simulink model "smceso_simscape"  (R2024a)
settings: Solver=VariableStepAuto  StartTime=0.0  StopTime=150  FixedStep=0.05  RelTol=1e-3  AbsTol=1e-3  EnableMultiTasking=on
model workspace (MATLAB code in the model file):
  | rCord = 0.25; % Cord radius, in
  | rho = 8000; % Density (steel), kg/m^3
  | 
  | % Hoist Pulleys:
  | rContactHoist = 7; % Contact radius, in
  | rPitchHoist = rContactHoist + rCord; % Pitch radius, in
  | Hoist.RGB = [0.35 0.35 1.0]; % Color, RGB 0-1
  | 
  | % Trolley Pulleys:
  | rContactTrolley = 5; % Contact radius, in
  | rPitchTrolley = rContactTrolley + rCord; % Pitch radius, in
  | Trolley.RGB = [1 0.15 0.15]; % Color, RGB 0-1
values from neighbouring files (symbols this model uses):
  m = 500    [finiteeso1.m]    (also in myIneqConFunction.m; robot_model.m)
  s = dq1 + lambda*(q1-q1d) + alpha*q2    [myIneqConFunction.m]
undefined symbols (not defined in the file or in its folder): X, Y, Z
libraries: sm_lib x19, nesl_utility x10
CloseFcn:
  | try,close(h1_sm_cable_tower_crane),end
  | clear h1_sm_cable_tower_crane
  | 
  | clear simlog_sm_cable_tower_crane
  | clear logsout_sm_cable_tower_crane
Description:
  | Tower Crane With Trolley and Hoist
settings Model: Creator=The MathWorks, Inc.  LastModifiedBy=vanch
settings SolverCC: AutoInsertRateTranBlk=on
settings DataIOCC: MaxDataPoints=10000  ReturnWorkspaceOutputs=off  SignalLoggingName=logsout_sm_cable_tower_crane
settings OptimizationCC: LifeSpan=inf
settings DebuggingCC: MultiTaskRateTransMsg=warning  UnconnectedInputMsg=warning  UnconnectedOutputMsg=warning  UnconnectedLineMsg=warning  AllowSymbolicDim=off  PregeneratedLibrarySubsystemCodeDiagnostic=none  SFUnexpectedBacktrackingDiag=warning  SFNoUnconditionalDefaultTransitionDiag=warning  SFExecutionAtInitializationDiag=none  ArithmeticOperatorsInVariantConditions=warning
settings ModelReferenceCC: EnableRefExpFcnMdlSchedulingChecks=on
settings SFSimCC: SimUseLocalCustomCode=off  CustomCodeUndefinedFunction=UseInterfaceOnly
settings RTWCC: RTWUseLocalCustomCode=off  GPUComputeCapability=3.5  DLArmComputeVersion=19.05
settings CodeAppCC: StateflowObjectComments=on
settings GRTTargetCC: TargetLangStandard=C89/C90 (ANSI)
settings ConfigComp: CovMetricSettings=dw  CovSaveCumulativeToWorkspaceVar=on  CovSaveSingleToWorkspaceVar=on  CovExternalEMLEnable=off  CovSFcnEnable=off
settings SimscapeCC: SimscapeNormalizeSystem=off  SimscapeLogType=all  SimscapeLogSimulationStatistics=on  SimscapeLogName=simlog_sm_cable_tower_crane  SimscapeLogDataHistory=10000
settings ConfigurationSet: Description=SimMechanics 2G
settings DiagnosticsConfigSet: SimMechanicsUnconnectedFramePorts=none
settings ExplorerConfigSet: InternalSimMechanicsExplorerSettings="<ExplorerConfiguration><canonicalview>default</canonicalview><AnimationSetting><BasePlaybackSpeed>1.0</BasePlaybackSpeed><PlaybackSpeedFactor>4.0</PlaybackSpeedFactor></AnimationSetting><TilePanel><TileInfo><Tiles Columns=\"2\" Count=\"3\" Rows=\"2\"><Column Weight=\"0.5346\"/><Column Weight=\"0.4654\"/><Row Weight=\"0.5103\"/><Row Weight=\"0.4897\"/><Tile Height=\"2\" Width=\"1\" X=\"0\" Y=\"0\"/><Tile Height=\"1\" Width=\"1\" X=\"1\" Y=\"0\"/><Tile Height=\"1\" Width=\"1\" X=\"1\" Y=\"1\"/></Tiles></TileInfo><SceneInfo><SceneViewer><BGColor><R>1</R><G>1</G><B>1</B></BGColor><Camera><DoPerspective>off</DoPerspective><Position><X>21.2245234512222218</X><Y>-52.6270053119242149</Y><Z>31.1052414476314176</Z></Position><Center><X>4.03969410390390138</X><Y>-11.531029179114606</Y><Z>26.0581003831327429</Z></Center><Up><X>-0.0463963572767632781</X><Y>0.102630781540790306</Y><Z>0.993636905872448795</Z></Up><ViewLimDist>1</ViewLimDist><YLim>29.3741015052795404</YLim><XLim>20.323349428569383</XLim></Camera></SceneViewer><SceneViewer><BGColor><R>1</R><G>1</G><B>1</B></BGColor><Camera><DoPerspective>on</DoPerspective><Position><X>7.62097636835298875</X><Y>-7.28765998656097835</Y><Z>48.5790735257936888</Z></Position><Center><X>8.43815474417762879</X><Y>-4.87266112484600811</Y><Z>48.0790735257936888</Z></Center><Up><X>-5.5511151231257827e-17</X><Y>5.5511151231257827e-16</Y><Z>1</Z></Up><ViewLimDist>1</ViewLimDist><YLim>0.466307658154998583</YLim><XLim>0.554639064765857337</XLim></Camera></SceneViewer><SceneViewer><BGColor><R>1</R><G>1</G><B>1</B></BGColor><Camera><DoPerspective>on</DoPerspective><Position><X>8.91771748690350918</X><Y>-5.72696404215155486</Y><Z>6.27537931293847695</Z></Position><Center><X>8.30176786249526799</X><Y>-4.79390373339482956</Y><Z>6.27750543949919315</Z></Center><Up><X>0.0018411954977133882</X><Y>-0.00106320895941669491</Y><Z>0.999997739790369544</Z></Up><ViewLimDist>1</ViewLimDist><YLim>0.466307658154998583</YLim><XLim>0.577537007806649627</XLim></Camera></SceneViewer></SceneInfo></TilePanel><MechEditorPanel><Cameras><Camera><Id>Camera3</Id><Value><Name>FrontPerspective</Name><NativeCamera><PositionKeyframeSet><Keyframe><Time>+0.0000000000000000e+00</Time><Value><X>-8.2854741987599496e+01</X><Y>+6.9234458953745950e+00</Y><Z>-1.4145124864096545e+01</Z></Value></Keyframe></PositionKeyframeSet><CenterKeyframeSet><Keyframe><Time>+0.0000000000000000e+00</Time><Value><X>-3.8386611818308438e+01</X><Y>+5.6305115971696154e+00</Y><Z>-1.4885098486593563e+01</Z></Value></Keyframe></CenterKeyframeSet><UpVectorKeyframeSet><Keyframe><Time>+0.0000000000000000e+00</Time><Value><X>+1.6618412601474140e-02</X><Y>-6.8180478671186931e-04</Y><Z>+9.9986167218512778e-01</Z></Value></Keyframe></UpVectorKeyframeSet></NativeCamera></Value></Camera><Camera><Id>Camera4</Id><Value><Name>IsoPerspective</Name><NativeCamera><PositionKeyframeSet><Keyframe><Time>+0.0000000000000000e+00</Time><Value><X>+4.8041868307394381e+01</X><Y>-7.2574542010436318e+01</Y><Z>-1.9623596137357460e+01</Z></Value></Keyframe></PositionKeyframeSet><CenterKeyframeSet><Keyframe><Time>+0.0000000000000000e+00</Time><Value><X>+1.8405017763935820e+01</X><Y>-3.4347633911723840e+01</Y><Z>-1.7683820531547433e+01</Z></Value></Keyframe></CenterKeyframeSet><UpVectorKeyframeSet><Keyframe><Time>+0.0000000000000000e+00</Time><Value><X>+2.6442579825491388e-02</X><Y>-3.0202215803021151e-02</Y><Z>+9.9919398323486741e-01</Z></Value></Keyframe></UpVectorKeyframeSet></NativeCamera></Value></Camera><Camera><Id>Camera5</Id><Value><Name>TrolleyCam</Name><NativeCamera><PositionTrackingFeature>Tower_Crane.Trolley.Transform_Trolley_Cam.F</PositionTrackingFeature><CenterTrackingFeature>Tower_Crane.Trolley.Trolley.R</CenterTrackingFeature><UpVectorTrackingFeature>Tower_Crane.Trolley.Trolley.R</UpVectorTrackingFeature><CenterTrackingOrigin>on</CenterTrackingOrigin><UpVectorTrackingDirection>+Y</UpVectorTrackingDirection></NativeCamera></Value></Camera><Camera><Id>Camera6</Id><Value><Name>BlockCam</Name><NativeCamera><PositionTrackingFeature>Tower_Crane.Hoist_Pulleys.Transform_Block_Cam.F</PositionTrackingFeature><CenterTrackingFeature>Tower_Crane.Hoist_Pulleys.Revolute_Block_Pulley.F</CenterTrackingFeature><UpVectorTrackingFeature>Tower_Crane.Hoist_Pulleys.Revolute_Block_Pulley.F</UpVectorTrackingFeature><CenterTrackingOrigin>on</CenterTrackingOrigin><UpVectorTrackingDirection>-Y</UpVectorTrackingDirection></NativeCamera></Value></Camera></Cameras><GfxPanelCameraMap><MapElement CameraMLId=\"Camera5\" GfxPanelIndex=\"1\"/><MapElement CameraMLId=\"Camera6\" GfxPanelIndex=\"2\"/></GfxPanelCameraMap><VideoCreator><PlaybackSpeedRatio>1.0</PlaybackSpeedRatio><FrameRate>30</FrameRate><VideoFormat>MPEG-4</VideoFormat><FrameSize>auto</FrameSize></VideoCreator></MechEditorPanel></ExplorerConfiguration>"

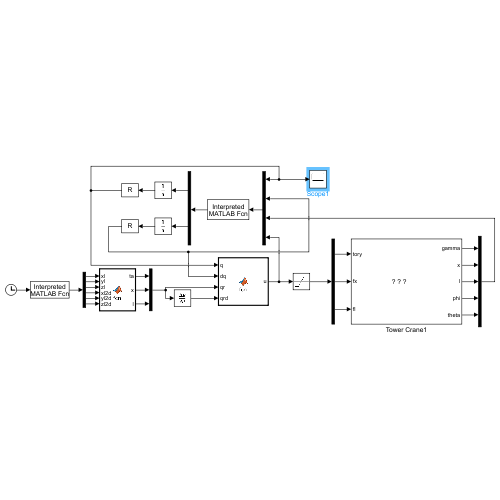
[thumbnail: Simulink's stored preview of the top-level diagram]
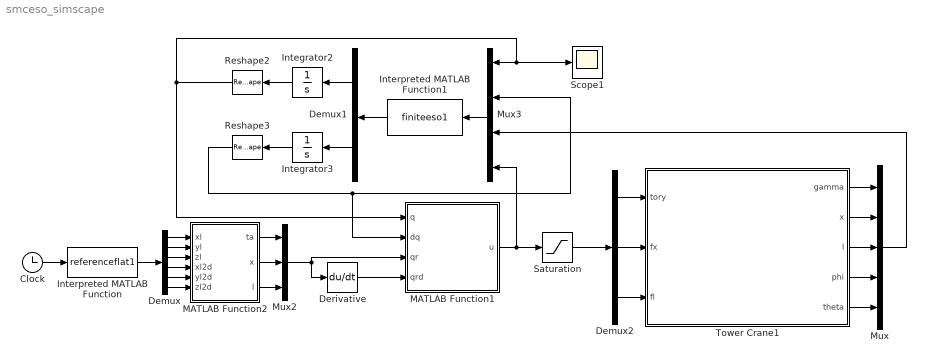
== system smceso_simscape ==
  Clock : Clock
  Demux : Demux  Outputs=6
  Demux1 : Demux  Outputs=2
  Demux2 : Demux  Outputs=3
  Derivative : Derivative
  Integrator2 : Integrator  InitialCondition=[0;0;45;0;0]
  Integrator3 : Integrator  InitialCondition=[0;0;0;0;0]
  Interpreted MATLAB Function : MATLABFcn  MATLABFcn=referenceflat1  OutputDimensions=6
  Interpreted MATLAB Function1 : MATLABFcn  MATLABFcn=finiteeso1
  MATLAB Function1 : MATLAB Function  TreatAsAtomicUnit=on
  MATLAB Function2 : MATLAB Function  TreatAsAtomicUnit=on
  Mux : Mux  Inputs=5
  Mux2 : Mux  Inputs=3
  Mux3 : Mux
  Reshape2 : Reshape  OutputDimensionality=Customize  OutputDimensions=[5,1]
  Reshape3 : Reshape  OutputDimensionality=Customize  OutputDimensions=[5,1]
  Saturation : Saturate  UpperLimit=[2000;400;0]  LowerLimit=[-2000;-400;-6000]
  Scope1 : Scope
  Tower Crane1 : Subsystem  Tag=PublishSubsystem
      mask Display: image('sm_cable_tower_crane_all_IMAGE.png');
  wires:
  Demux2/1 -> Tower Crane1/1(tory)
  Demux2/2 -> Tower Crane1/2(fx)
  Demux2/3 -> Tower Crane1/3(fl)
  Clock/1 -> Interpreted MATLAB Function/1
  Mux2/1 -> Derivative/1, MATLAB Function1/3(qr)
  MATLAB Function2/1(ta) -> Mux2/1
  Mux/1 -> Mux3/3
  Demux/4 -> MATLAB Function2/4(xl2d)
  Demux/3 -> MATLAB Function2/3(zl)
  Mux3/1 -> Interpreted MATLAB Function1/1
  Demux1/2 -> Integrator3/1
  Derivative/1 -> MATLAB Function1/4(qrd)
  MATLAB Function2/2(x) -> Mux2/2
  Interpreted MATLAB Function/1 -> Demux/1
  Integrator2/1 -> Reshape2/1
  Reshape3/1 -> Mux3/2, MATLAB Function1/2(dq)
  Integrator3/1 -> Reshape3/1
  Interpreted MATLAB Function1/1 -> Demux1/1
  Reshape2/1 -> Scope1/1, Mux3/1, MATLAB Function1/1(q)
  Demux/5 -> MATLAB Function2/5(yl2d)
  MATLAB Function2/3(l) -> Mux2/3
  Demux/6 -> MATLAB Function2/6(zl2d)
  Demux/1 -> MATLAB Function2/1(xl)
  MATLAB Function1/1(u) -> Saturation/1, Mux3/4
  Demux/2 -> MATLAB Function2/2(yl)
  Demux1/1 -> Integrator2/1
  Tower Crane1/1(gamma) -> Mux/1
  Tower Crane1/2(x) -> Mux/2
  Tower Crane1/3(l) -> Mux/3
  Tower Crane1/4(phi) -> Mux/4
  Tower Crane1/5(theta) -> Mux/5
  Saturation/1 -> Demux2/1

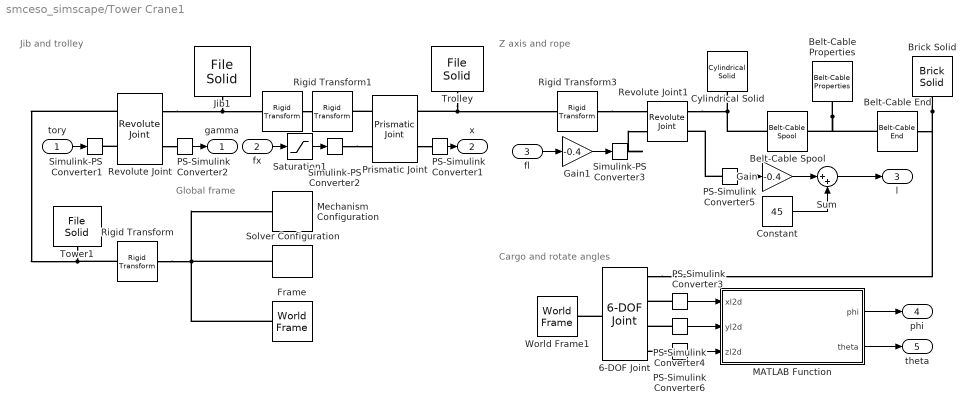
== system smceso_simscape/Tower Crane1 ==
  note: Z axis and rope
  note: Cargo and rotate
      | angles
  note: Jib and trolley
  note: Global frame
  tory : Inport
  fx : Inport  Port=2
  fl : Inport  Port=3
  " Frame" : sm_lib/Frames and Transforms/World Frame
  " " : sm_lib/Frames and Transforms/Rigid Transform  RotationMethod=StandardAxis  FollAlignAxisA=+X  BaseAlignAxisA=+Y  FollAlignAxisB=+Y  BaseAlignAxisB=+Z  RotationStandardAxis=+X  RotationAngle=90  RotationAngleUnits=deg  RotationArbitraryAxis=[0 0 1]  RotationSequenceAxes=FollowerAxes  RotationSequence=XYX  RotationSequenceAngles=[0 0 0]  RotationSequenceAnglesUnits=deg  RotationMatrix=[1 0 0; 0 1 0; 0 0 1]  Quaternion=[1 0 0 0]  TranslationMethod=StandardAxis  TranslationCartesianOffset=[-2.5 0.5 0.5]  TranslationCartesianOffsetUnits=m  TranslationStandardAxis=+Y  TranslationStandardOffset=3.2  TranslationStandardOffsetUnits=m  TranslationROffset=0  TranslationROffsetUnits=m  TranslationThetaOffset=0  TranslationThetaOffsetUnits=deg  TranslationZOffset=0  TranslationZOffsetUnits=m
  6-DOF Joint : sm_lib/Joints/6-DOF Joint  JointMode=Normal  CompositeWrenchDir=FollowerOnBase  CompositeWrenchFrame=BaseFrame  SenseConstraintForce=off  SenseConstraintTorque=off  SenseTotalForce=off  SenseTotalTorque=off  PxPositionTargetSpecify=on  PxPositionTargetPriority=High  PxPositionTargetValue=-6  PxPositionTargetValueUnits=m  PxVelocityTargetSpecify=off  PxVelocityTargetPriority=High  PxVelocityTargetValue=0  PxVelocityTargetValueUnits=m/s  PxEquilibriumPosition=0  PxEquilibriumPositionUnits=m  PxSpringStiffness=0  PxSpringStiffnessUnits=N/m  PxDampingCoefficient=0  PxDampingCoefficientUnits=N/(m/s)  PxLowerLimitSpecify=off  PxLowerLimitBound=-1  PxLowerLimitBoundUnits=m  PxLowerLimitStiffness=1e6  PxLowerLimitStiffnessUnits=N/m  PxLowerLimitDamping=1e3  PxLowerLimitDampingUnits=N/(m/s)  PxLowerLimitTransitionRegionWidth=1e-4  PxLowerLimitTransitionRegionWidthUnits=m  PxUpperLimitSpecify=off  PxUpperLimitBound=1  PxUpperLimitBoundUnits=m  PxUpperLimitStiffness=1e6  PxUpperLimitStiffnessUnits=N/m  PxUpperLimitDamping=1e3  PxUpperLimitDampingUnits=N/(m/s)  PxUpperLimitTransitionRegionWidth=1e-4  PxUpperLimitTransitionRegionWidthUnits=m  PxTorqueActuationMode=NoTorque  PxMotionActuationMode=ComputedMotion  PxSensePosition=off  PxSenseVelocity=off  PxSenseAcceleration=on  PxSenseTorqueForce=off  PxSenseLowerLimitTorqueForce=off  PxSenseUpperLimitTorqueForce=off  PyPositionTargetSpecify=on  PyPositionTargetPriority=High  PyPositionTargetValue=0  PyPositionTargetValueUnits=m  PyVelocityTargetSpecify=off  PyVelocityTargetPriority=High  PyVelocityTargetValue=0  PyVelocityTargetValueUnits=m/s  PyEquilibriumPosition=0  PyEquilibriumPositionUnits=m  PySpringStiffness=0  PySpringStiffnessUnits=N/m  PyDampingCoefficient=0  PyDampingCoefficientUnits=N/(m/s)  PyLowerLimitSpecify=off  PyLowerLimitBound=-1  PyLowerLimitBoundUnits=m  PyLowerLimitStiffness=1e6  PyLowerLimitStiffnessUnits=N/m  PyLowerLimitDamping=1e3  PyLowerLimitDampingUnits=N/(m/s)  PyLowerLimitTransitionRegionWidth=1e-4  PyLowerLimitTransitionRegionWidthUnits=m  PyUpperLimitSpecify=off  PyUpperLimitBound=1  PyUpperLimitBoundUnits=m  PyUpperLimitStiffness=1e6  PyUpperLimitStiffnessUnits=N/m  PyUpperLimitDamping=1e3  PyUpperLimitDampingUnits=N/(m/s)  PyUpperLimitTransitionRegionWidth=1e-4  PyUpperLimitTransitionRegionWidthUnits=m  PyTorqueActuationMode=NoTorque  PyMotionActuationMode=ComputedMotion  PySensePosition=off  PySenseVelocity=off  PySenseAcceleration=on  PySenseTorqueForce=off  PySenseLowerLimitTorqueForce=off  PySenseUpperLimitTorqueForce=off  PzPositionTargetSpecify=on  PzPositionTargetPriority=High  PzPositionTargetValue=3  PzPositionTargetValueUnits=m  PzVelocityTargetSpecify=off  PzVelocityTargetPriority=High  PzVelocityTargetValue=0  PzVelocityTargetValueUnits=m/s  PzEquilibriumPosition=0  PzEquilibriumPositionUnits=m  PzSpringStiffness=0  PzSpringStiffnessUnits=N/m  PzDampingCoefficient=30  PzDampingCoefficientUnits=N/(m/s)  PzLowerLimitSpecify=off  PzLowerLimitBound=-1  PzLowerLimitBoundUnits=m  PzLowerLimitStiffness=1e6  PzLowerLimitStiffnessUnits=N/m  PzLowerLimitDamping=1e3  PzLowerLimitDampingUnits=N/(m/s)  PzLowerLimitTransitionRegionWidth=1e-4  PzLowerLimitTransitionRegionWidthUnits=m  PzUpperLimitSpecify=off  PzUpperLimitBound=1  PzUpperLimitBoundUnits=m  PzUpperLimitStiffness=1e6  PzUpperLimitStiffnessUnits=N/m  PzUpperLimitDamping=1e3  PzUpperLimitDampingUnits=N/(m/s)  PzUpperLimitTransitionRegionWidth=1e-4  PzUpperLimitTransitionRegionWidthUnits=m  PzTorqueActuationMode=NoTorque  PzMotionActuationMode=ComputedMotion  PzSensePosition=off  PzSenseVelocity=off  PzSenseAcceleration=on  PzSenseTorqueForce=off  PzSenseLowerLimitTorqueForce=off  PzSenseUpperLimitTorqueForce=off  SphPositionTargetSpecify=off  SphPositionTargetPriority=High  SphPositionTargetRotationMethod=None  SphPositionTargetFollAlignAxisA=+X  SphPositionTargetBaseAlignAxisA=+Y  SphPositionTargetFollAlignAxisB=+Y  SphPositionTargetBaseAlignAxisB=+Z  SphPositionTargetRotationStandardAxis=+Z  SphPositionTargetRotationAngle=0.0  SphPositionTargetRotationAngleUnits=deg  SphPositionTargetRotationArbitraryAxis=[0 0 1]  SphPositionTargetRotationSequenceAxes=FollowerAxes  SphPositionTargetRotationSequence=XYX  SphPositionTargetRotationSequenceAngles=[0 0 0]  SphPositionTargetRotationSequenceAnglesUnits=deg  SphPositionTargetRotationMatrix=[1 0 0; 0 1 0; 0 0 1]  SphPositionTargetQuaternion=[1 0 0 0]  SphVelocityTargetSpecify=off  SphVelocityTargetPriority=High  SphVelocityTargetValue=[0 0 0]  SphVelocityTargetValueUnits=deg/s  SphVelocityTargetInFollowerFrame=on  SphEqPosRotationMethod=None  SphEqPosFollAlignAxisA=+X  SphEqPosBaseAlignAxisA=+Y  SphEqPosFollAlignAxisB=+Y  SphEqPosBaseAlignAxisB=+Z  SphEqPosRotationStandardAxis=+Z  SphEqPosRotationAngle=0.0  SphEqPosRotationAngleUnits=deg  SphEqPosRotationArbitraryAxis=[0 0 1]  SphEqPosRotationSequenceAxes=FollowerAxes  SphEqPosRotationSequence=XYX  SphEqPosRotationSequenceAngles=[0 0 0]  SphEqPosRotationSequenceAnglesUnits=deg  SphEqPosRotationMatrix=[1 0 0; 0 1 0; 0 0 1]  SphEqPosQuaternion=[1 0 0 0]  SphSpringStiffness=0  SphSpringStiffnessUnits=N*m/deg  SphDampingCoefficient=0  SphDampingCoefficientUnits=N*m/(deg/s)  SphLowerLimitSpecify=off  SphLowerLimitBound=15  SphLowerLimitBoundUnits=deg  SphLowerLimitStiffness=1e4  SphLowerLimitStiffnessUnits=N*m/deg  SphLowerLimitDamping=10  SphLowerLimitDampingUnits=N*m/(deg/s)  SphLowerLimitTransitionRegionWidth=0.1  SphLowerLimitTransitionRegionWidthUnits=deg  SphUpperLimitSpecify=off  SphUpperLimitBound=45  SphUpperLimitBoundUnits=deg  SphUpperLimitStiffness=1e4  SphUpperLimitStiffnessUnits=N*m/deg  SphUpperLimitDamping=10  SphUpperLimitDampingUnits=N*m/(deg/s)  SphUpperLimitTransitionRegionWidth=0.1  SphUpperLimitTransitionRegionWidthUnits=deg  SphTorqueActuationMode=NoTorque  SphActuateTorqueX=off  SphActuateTorqueY=off  SphActuateTorqueZ=off  SphActuateTorque=off  SphActuationFrame=BaseFrame  SphSensePosition=off  SphSenseVelocityX=off  SphSenseVelocityY=off  SphSenseVelocityZ=off  SphSenseVelocity=off  SphSenseAccelerationX=off  SphSenseAccelerationY=off  SphSenseAccelerationZ=off  SphSenseAcceleration=off  SphSenseLowerLimitTorqueMag=off  SphSenseUpperLimitTorqueMag=off  SphSensingFrame=BaseFrame
  Belt-Cable Properties : sm_lib/Belts and Cables/Belt-Cable Properties  DrumBeltCableAlignment=Unrestricted  GraphicType=PitchLine  GraphicVisPropType=SimpleVisualProperties  GraphicDiffuseColor=[0.5 0.5 0.5]  GraphicOpacity=1.0  GraphicSpecularColor=[0.5 0.5 0.5 1.0]  GraphicAmbientColor=[0.15 0.15 0.15 1.0]  GraphicEmissiveColor=[0.0 0.0 0.0 1.0]  GraphicShininess=75
  Belt-Cable End : sm_lib/Belts and Cables/Belt-Cable End
  Belt-Cable Spool : sm_lib/Belts and Cables/Belt-Cable Spool  PitchRadius=0.4  PitchRadiusUnits=m  SenseSpoolAngleA=off  SenseFleetAngleA=off
  Brick Solid : sm_lib/Body Elements/Brick Solid  BrickDimensions=[1 1 1]  BrickDimensionsUnits=m  ExportEntireGeometry=off  InertiaType=CalculateFromGeometry  BasedOnType=Density  Density=500  DensityUnits=kg/m^3  Mass=1  MassUnits=kg  CenterOfMass=[0 0 0]  CenterOfMassUnits=m  MomentsOfInertia=[1 1 1]  MomentsOfInertiaUnits=kg*m^2  ProductsOfInertia=[0 0 0]  ProductsOfInertiaUnits=kg*m^2  GraphicType=FromGeometry  MarkerShape=Sphere  MarkerSize=10  GraphicVisPropType=SimpleVisualProperties  GraphicDiffuseColor=[0.5 0.5 0.5]  GraphicOpacity=1.0  GraphicSpecularColor=[0.5 0.5 0.5 1.0]  GraphicAmbientColor=[0.15 0.15 0.15 1.0]  GraphicEmissiveColor=[0.0 0.0 0.0 1.0]  GraphicShininess=75  DoExposeReferenceFrame=on  SerializedFrames=<Frames/>
  Constant : Constant  Value=45
  Cylindrical Solid : sm_lib/Body Elements/Cylindrical Solid  CylinderRadius=0.5  CylinderRadiusUnits=m  CylinderLength=0.4  CylinderLengthUnits=m  ExportEntireGeometry=off  InertiaType=CalculateFromGeometry  BasedOnType=Density  Density=1000  DensityUnits=kg/m^3  Mass=1  MassUnits=kg  CenterOfMass=[0 0 0]  CenterOfMassUnits=m  MomentsOfInertia=[1 1 1]  MomentsOfInertiaUnits=kg*m^2  ProductsOfInertia=[0 0 0]  ProductsOfInertiaUnits=kg*m^2  GraphicType=FromGeometry  MarkerShape=Sphere  MarkerSize=10  GraphicVisPropType=SimpleVisualProperties  GraphicDiffuseColor=[0.5 0.5 0.5]  GraphicOpacity=1.0  GraphicSpecularColor=[0.5 0.5 0.5 1.0]  GraphicAmbientColor=[0.15 0.15 0.15 1.0]  GraphicEmissiveColor=[0.0 0.0 0.0 1.0]  GraphicShininess=75  DoExposeReferenceFrame=on  SerializedFrames=<Frames/>
  Gain : Gain  Gain=-0.4
  Gain1 : Gain  Gain=-0.4
  Jib1 : sm_lib/Body Elements/File Solid  ExtGeomFileName=jib.step  UnitType=FromFile  ExtGeomFileUnits=m  StepReaderType=HEX  ExportConvexHullGeometry=off  InertiaType=CalculateFromGeometry  BasedOnType=Density  Density=400  DensityUnits=kg/(m^3)  Mass=1  MassUnits=kg  CenterOfMass=[0 0 0]  CenterOfMassUnits=m  MomentsOfInertia=[1 1 1]  MomentsOfInertiaUnits=kg*m^2  ProductsOfInertia=[0 0 0]  ProductsOfInertiaUnits=kg*m^2  GraphicType=FromGeometry  MarkerShape=Sphere  MarkerSize=10  GraphicVisPropType=AdvancedVisualProperties  GraphicDiffuseColor=[0.15 0.15 0.15]  GraphicOpacity=1.0  GraphicSpecularColor=[0.6 0.6 0.6]  GraphicAmbientColor=[0.1 0.1 0.1]  GraphicEmissiveColor=[0.0 0.0 0.0 1.0]  GraphicShininess=10  DoExposeReferenceFrame=on  SerializedFrames=<Frames/>
  MATLAB Function : MATLAB Function  TreatAsAtomicUnit=on
  Mechanism Configuration : sm_lib/Utilities/Mechanism Configuration  UniformGravity=Constant  GravityVector=[0 0 -9.81]  GravityVectorUnits=m/s^2  LinearizationDelta=0.001  JointModeTransitionNonlinearIterations=2
  PS-Simulink Converter{1..6} (6 alike) : nesl_utility/PS-Simulink Converter  PhysicalDomain=network_engine_domain  SubClassName=ps_output  LeftPortType=input  RightPortType=output  PseudoPeriodic=off  Frequencies=[]  VectorFormat=inherit  Unit=inherit  AffineConversion=off
  Prismatic Joint : sm_lib/Joints/Prismatic Joint  JointMode=Normal  CompositeWrenchDir=FollowerOnBase  CompositeWrenchFrame=BaseFrame  SenseConstraintForce=off  SenseConstraintTorque=off  SenseTotalForce=off  SenseTotalTorque=off  PositionTargetSpecify=off  PositionTargetPriority=High  PositionTargetValue=0  PositionTargetValueUnits=m  VelocityTargetSpecify=off  VelocityTargetPriority=High  VelocityTargetValue=0  VelocityTargetValueUnits=m/s  EquilibriumPosition=0  EquilibriumPositionUnits=m  SpringStiffness=0  SpringStiffnessUnits=N/m  DampingCoefficient=50  DampingCoefficientUnits=N/(m/s)  LowerLimitSpecify=off  LowerLimitBound=-1  LowerLimitBoundUnits=m  LowerLimitStiffness=1e6  LowerLimitStiffnessUnits=N/m  LowerLimitDamping=1e3  LowerLimitDampingUnits=N/(m/s)  LowerLimitTransitionRegionWidth=1e-4  LowerLimitTransitionRegionWidthUnits=m  UpperLimitSpecify=off  UpperLimitBound=1  UpperLimitBoundUnits=m  UpperLimitStiffness=1e6  UpperLimitStiffnessUnits=N/m  UpperLimitDamping=1e3  UpperLimitDampingUnits=N/(m/s)  UpperLimitTransitionRegionWidth=1e-4  UpperLimitTransitionRegionWidthUnits=m  TorqueActuationMode=InputTorque  MotionActuationMode=ComputedMotion  SensePosition=on  SenseVelocity=off  SenseAcceleration=off  SenseTorqueForce=off  SenseLowerLimitTorqueForce=off  SenseUpperLimitTorqueForce=off
  Revolute Joint : sm_lib/Joints/Revolute Joint  JointMode=Normal  CompositeWrenchDir=FollowerOnBase  CompositeWrenchFrame=BaseFrame  SenseConstraintForce=off  SenseConstraintTorque=off  SenseTotalForce=off  SenseTotalTorque=off  PositionTargetSpecify=off  PositionTargetPriority=High  PositionTargetValue=0  PositionTargetValueUnits=deg  VelocityTargetSpecify=off  VelocityTargetPriority=High  VelocityTargetValue=0  VelocityTargetValueUnits=deg/s  EquilibriumPosition=0  EquilibriumPositionUnits=deg  SpringStiffness=0  SpringStiffnessUnits=N*m/deg  DampingCoefficient=30  DampingCoefficientUnits=N*m/(deg/s)  LowerLimitSpecify=off  LowerLimitBound=-90  LowerLimitBoundUnits=deg  LowerLimitStiffness=1e4  LowerLimitStiffnessUnits=N*m/deg  LowerLimitDamping=10  LowerLimitDampingUnits=N*m/(deg/s)  LowerLimitTransitionRegionWidth=0.1  LowerLimitTransitionRegionWidthUnits=deg  UpperLimitSpecify=off  UpperLimitBound=90  UpperLimitBoundUnits=deg  UpperLimitStiffness=1e4  UpperLimitStiffnessUnits=N*m/deg  UpperLimitDamping=10  UpperLimitDampingUnits=N*m/(deg/s)  UpperLimitTransitionRegionWidth=0.1  UpperLimitTransitionRegionWidthUnits=deg  TorqueActuationMode=InputTorque  MotionActuationMode=ComputedMotion  SensePosition=on  SenseVelocity=off  SenseAcceleration=off  SenseTorqueForce=off  SenseLowerLimitTorqueForce=off  SenseUpperLimitTorqueForce=off
  Revolute Joint1 : sm_lib/Joints/Revolute Joint  JointMode=Normal  CompositeWrenchDir=FollowerOnBase  CompositeWrenchFrame=FollowerFrame  SenseConstraintForce=off  SenseConstraintTorque=off  SenseTotalForce=off  SenseTotalTorque=off  PositionTargetSpecify=off  PositionTargetPriority=High  PositionTargetValue=0  PositionTargetValueUnits=deg  VelocityTargetSpecify=off  VelocityTargetPriority=High  VelocityTargetValue=0  VelocityTargetValueUnits=deg/s  EquilibriumPosition=0  EquilibriumPositionUnits=deg  SpringStiffness=0  SpringStiffnessUnits=N*m/deg  DampingCoefficient=0  DampingCoefficientUnits=N*m/(deg/s)  LowerLimitSpecify=off  LowerLimitBound=-90  LowerLimitBoundUnits=deg  LowerLimitStiffness=1e4  LowerLimitStiffnessUnits=N*m/deg  LowerLimitDamping=10  LowerLimitDampingUnits=N*m/(deg/s)  LowerLimitTransitionRegionWidth=0.1  LowerLimitTransitionRegionWidthUnits=deg  UpperLimitSpecify=off  UpperLimitBound=90  UpperLimitBoundUnits=deg  UpperLimitStiffness=1e4  UpperLimitStiffnessUnits=N*m/deg  UpperLimitDamping=10  UpperLimitDampingUnits=N*m/(deg/s)  UpperLimitTransitionRegionWidth=0.1  UpperLimitTransitionRegionWidthUnits=deg  TorqueActuationMode=InputTorque  MotionActuationMode=ComputedMotion  SensePosition=on  SenseVelocity=off  SenseAcceleration=off  SenseTorqueForce=off  SenseLowerLimitTorqueForce=off  SenseUpperLimitTorqueForce=off
  Rigid Transform : sm_lib/Frames and Transforms/Rigid Transform  RotationMethod=None  FollAlignAxisA=+X  BaseAlignAxisA=+Y  FollAlignAxisB=+Y  BaseAlignAxisB=+Z  RotationStandardAxis=+Z  RotationAngle=0.0  RotationAngleUnits=deg  RotationArbitraryAxis=[0 0 1]  RotationSequenceAxes=FollowerAxes  RotationSequence=XYX  RotationSequenceAngles=[0 0 0]  RotationSequenceAnglesUnits=deg  RotationMatrix=[1 0 0; 0 1 0; 0 0 1]  Quaternion=[1 0 0 0]  TranslationMethod=StandardAxis  TranslationCartesianOffset=[0 0 0]  TranslationCartesianOffsetUnits=m  TranslationStandardAxis=+Z  TranslationStandardOffset=43.375  TranslationStandardOffsetUnits=m  TranslationROffset=0  TranslationROffsetUnits=m  TranslationThetaOffset=0  TranslationThetaOffsetUnits=deg  TranslationZOffset=0  TranslationZOffsetUnits=m
  Rigid Transform1 : sm_lib/Frames and Transforms/Rigid Transform  RotationMethod=StandardAxis  FollAlignAxisA=+X  BaseAlignAxisA=+Y  FollAlignAxisB=+Y  BaseAlignAxisB=+Z  RotationStandardAxis=-Y  RotationAngle=90  RotationAngleUnits=deg  RotationArbitraryAxis=[0 0 1]  RotationSequenceAxes=FollowerAxes  RotationSequence=XYX  RotationSequenceAngles=[0 0 0]  RotationSequenceAnglesUnits=deg  RotationMatrix=[1 0 0; 0 1 0; 0 0 1]  Quaternion=[1 0 0 0]  TranslationMethod=StandardAxis  TranslationCartesianOffset=[0 0 0]  TranslationCartesianOffsetUnits=m  TranslationStandardAxis=-X  TranslationStandardOffset=6  TranslationStandardOffsetUnits=m  TranslationROffset=0  TranslationROffsetUnits=m  TranslationThetaOffset=0  TranslationThetaOffsetUnits=deg  TranslationZOffset=0  TranslationZOffsetUnits=m
  Rigid Transform3 : sm_lib/Frames and Transforms/Rigid Transform  RotationMethod=StandardAxis  FollAlignAxisA=+X  BaseAlignAxisA=+Y  FollAlignAxisB=+Y  BaseAlignAxisB=+Z  RotationStandardAxis=+Z  RotationAngle=90  RotationAngleUnits=deg  RotationArbitraryAxis=[0 0 1]  RotationSequenceAxes=FollowerAxes  RotationSequence=XYX  RotationSequenceAngles=[0 0 0]  RotationSequenceAnglesUnits=deg  RotationMatrix=[1 0 0; 0 1 0; 0 0 1]  Quaternion=[1 0 0 0]  TranslationMethod=StandardAxis  TranslationCartesianOffset=[0 0 0]  TranslationCartesianOffsetUnits=m  TranslationStandardAxis=-Z  TranslationStandardOffset=0.4  TranslationStandardOffsetUnits=m  TranslationROffset=0  TranslationROffsetUnits=m  TranslationThetaOffset=0  TranslationThetaOffsetUnits=deg  TranslationZOffset=0  TranslationZOffsetUnits=m
  Saturation1 : Saturate  UpperLimit=100  LowerLimit=-100
  Simulink-PS Converter1 : nesl_utility/Simulink-PS Converter  PhysicalDomain=network_engine_domain  SubClassName=ps_input  LeftPortType=input  RightPortType=output  PseudoPeriodic=off  Frequencies=[]  NoiseDistribution=none  NoiseParameters=[]  Unit=1  AffineConversion=off  FilteringAndDerivatives=provide  SimscapeFilterOrder=1  InputFilterTimeConstant=0.001  UdotUserProvided=0
  Simulink-PS Converter2 : nesl_utility/Simulink-PS Converter  PhysicalDomain=network_engine_domain  SubClassName=ps_input  LeftPortType=input  RightPortType=output  PseudoPeriodic=off  Frequencies=[]  NoiseDistribution=none  NoiseParameters=[]  Unit=1  AffineConversion=off  FilteringAndDerivatives=provide  SimscapeFilterOrder=1  InputFilterTimeConstant=0.001  UdotUserProvided=0
  Simulink-PS Converter3 : nesl_utility/Simulink-PS Converter  PhysicalDomain=network_engine_domain  SubClassName=ps_input  LeftPortType=input  RightPortType=output  PseudoPeriodic=off  Frequencies=[]  NoiseDistribution=none  NoiseParameters=[]  Unit=1  AffineConversion=off  FilteringAndDerivatives=provide  SimscapeFilterOrder=1  InputFilterTimeConstant=0.001  UdotUserProvided=0
  Solver Configuration : nesl_utility/Solver Configuration  PhysicalDomain=network_engine_domain  SubClassName=solver  LeftPortType=input  RightPortType=generic  Tones=[]  Harmonics=[]  SimulateNoise=off  Profile=off  UseLocalSampling=off  EnableSwitchedLinearOptims=on  FrequencyDomain=off  UseCCode=off  RelTol=0.001  AbsTol=1e-06  MinStep=1e-09  ToWorkspace=off  RevertToSquareIcSolve=off  NumHomotopyIterations=100  PhasorMode=off  PhasorModeNumHarmonics=1  ConsistencySolver=NEWTON_FTOL  IndexReductionMethod=DerivativeReplacement  DoDC=off  ResidualTolerance=1e-09  ConsistencyTolSource=GLOBAL  ConsistencyAbsTol=0.001  ConsistencyRelTol=0.001  ConsistencyTolFactor=0.001  UseLocalSolver=off  LocalSolverChoice=NE_BACKWARD_EULER_ADVANCER  ResolveIndetEquations=on  FunctionEvalNumThread=1  LocalSolverSampleTime=0.001  DoFixedCost=off  MaxNonlinIter=3  MaxModeIter=2  ComputeImpulses=off  ImpulseIterations=1  LinearAlgebra=Sparse  LinearAlgebraNumThread=0  EquationFormulation=NE_TIME_EF  DelaysMemoryBudget=1024  AutomaticFiltering=on  FilteringTimeConstant=0.001  PartitionStorageMethod=AS_NEEDED  PartitionMemoryBudget=1024  PartitionMethod=FAST  MultibodyUseLocalSolver=off  MultibodyLocalSolverChoice=ODE1  MultibodyLocalSolverSampleTime=0.001
  Sum : Sum  Inputs=|++
  Tower1 : sm_lib/Body Elements/File Solid  ExtGeomFileName=tower.step  UnitType=FromFile  ExtGeomFileUnits=m  StepReaderType=HEX  ExportConvexHullGeometry=off  InertiaType=CalculateFromGeometry  BasedOnType=Density  Density=rho  DensityUnits=kg/(m^3)  Mass=1  MassUnits=kg  CenterOfMass=[0 0 0]  CenterOfMassUnits=m  MomentsOfInertia=[1 1 1]  MomentsOfInertiaUnits=kg*m^2  ProductsOfInertia=[0 0 0]  ProductsOfInertiaUnits=kg*m^2  GraphicType=FromGeometry  MarkerShape=Sphere  MarkerSize=10  GraphicVisPropType=AdvancedVisualProperties  GraphicDiffuseColor=[1.0 0.75 0.05]  GraphicOpacity=1.0  GraphicSpecularColor=[0.6 0.6 0.6]  GraphicAmbientColor=[0.1 0.1 0.1]  GraphicEmissiveColor=[0.0 0.0 0.0 1.0]  GraphicShininess=10  DoExposeReferenceFrame=on  SerializedFrames=<Frames/>
  "Trolley " : sm_lib/Body Elements/File Solid  ExtGeomFileName=trolley.step  UnitType=FromFile  ExtGeomFileUnits=m  StepReaderType=HEX  ExportConvexHullGeometry=off  InertiaType=CalculateFromGeometry  BasedOnType=Density  Density=7800  DensityUnits=kg/(m^3)  Mass=1  MassUnits=kg  CenterOfMass=[0 0 0]  CenterOfMassUnits=m  MomentsOfInertia=[1 1 1]  MomentsOfInertiaUnits=kg*m^2  ProductsOfInertia=[0 0 0]  ProductsOfInertiaUnits=kg*m^2  GraphicType=FromGeometry  MarkerShape=Sphere  MarkerSize=10  GraphicVisPropType=AdvancedVisualProperties  GraphicDiffuseColor=[1 0.75 0.05]  GraphicOpacity=1.0  GraphicSpecularColor=[0.4 0.4 0.4]  GraphicAmbientColor=[0 0 0]  GraphicEmissiveColor=[0 0 0]  GraphicShininess=10  DoExposeReferenceFrame=on  SerializedFrames=<Frames/>
  World Frame1 : sm_lib/Frames and Transforms/World Frame
  gamma : Outport
  x : Outport  Port=2
  l : Outport  Port=3
  phi : Outport  Port=4
  theta : Outport  Port=5
  wires:
  Gain1/1 -> Simulink-PS Converter3/1
  PS-Simulink Converter1/1 -> x/1
  PS-Simulink Converter2/1 -> gamma/1
  PS-Simulink Converter5/1 -> Gain/1
  fx/1 -> Saturation1/1
  Gain/1 -> Sum/1
  Sum/1 -> l/1
  Constant/1 -> Sum/2
  fl/1 -> Gain1/1
  tory/1 -> Simulink-PS Converter1/1
  Saturation1/1 -> Simulink-PS Converter2/1
  MATLAB Function/1(phi) -> phi/1
  MATLAB Function/2(theta) -> theta/1
  PS-Simulink Converter3/1 -> MATLAB Function/1(xl2d)
  PS-Simulink Converter4/1 -> MATLAB Function/2(yl2d)
  PS-Simulink Converter6/1 -> MATLAB Function/3(zl2d)
  connections:
  " "/LConn1 -- Rigid Transform1/LConn1
  Solver Configuration/RConn1 -- Mechanism Configuration/RConn1 -- Rigid Transform/LConn1 -- " Frame"/RConn1
  "Trolley "/RConn1 -- Prismatic Joint/RConn1 -- Rigid Transform3/LConn1
  Prismatic Joint/LConn1 -- Rigid Transform1/RConn1
  Simulink-PS Converter2/RConn1 -- Prismatic Joint/LConn2
  Tower1/RConn1 -- Revolute Joint/LConn1 -- Rigid Transform/RConn1
  Revolute Joint/LConn2 -- Simulink-PS Converter1/RConn1
  Jib1/RConn1 -- Revolute Joint/RConn1 -- " "/RConn1
  Belt-Cable Spool/LConn1 -- Revolute Joint1/RConn1 -- Cylindrical Solid/RConn1
  Brick Solid/RConn1 -- 6-DOF Joint/RConn1 -- Belt-Cable End/LConn1
  Belt-Cable Properties/LConn1 -- Belt-Cable End/RConn1 -- Belt-Cable Spool/RConn1
  Simulink-PS Converter3/RConn1 -- Revolute Joint1/LConn2
  Rigid Transform3/RConn1 -- Revolute Joint1/LConn1
  6-DOF Joint/LConn1 -- World Frame1/RConn1
  Prismatic Joint/RConn2 -- PS-Simulink Converter1/LConn1
  Revolute Joint/RConn2 -- PS-Simulink Converter2/LConn1
  PS-Simulink Converter5/LConn1 -- Revolute Joint1/RConn2
  PS-Simulink Converter3/LConn1 -- 6-DOF Joint/RConn2
  PS-Simulink Converter4/LConn1 -- 6-DOF Joint/RConn3
  PS-Simulink Converter6/LConn1 -- 6-DOF Joint/RConn4

== matlab function smceso_simscape/MATLAB Function1 ==
  data: q input; u output; dq input; qr input; qrd input
function u  = fcn(q, dq, qr,qrd)

mt=1140.7556;
j0=10215;
m=500;
bta=40;
bx=50;
bl=30;
btx=15;
bty=15;
g=9.81;

ta=q(1);
x=q(2);
l=q(3);
tx=q(4);
ty=q(5);
dta=dq(1);
dx=dq(2);
dl=dq(3);
dtx=dq(4);
dty=dq(5);
qa=[q(1);q(2);q(3)];
dqa=[dq(1);dq(2);dq(3)];
qu=[q(4);q(5)];
dqu=[dq(4);dq(5)];
e1=qa-qr;
e1d=dqa-qrd;
e2=[q(4);q(5)];

m11=j0+m*x^2+mt*x^2+m*l^2-m*l^2*cos(tx)^2*cos(ty)^2+2*m*x*l*cos(ty)*sin(tx);
m12=-m*l*sin(ty);
m13=m*x*sin(ty);
m14=-m*l^2*cos(tx)*cos(ty)*sin(ty);
m15=m*l^2*sin(tx)+m*x*l*cos(ty);
m21=-m*l*sin(ty);
m22=mt+m;
m23=m*cos(ty)*sin(tx);
m24=m*l*cos(tx)*cos(ty);
m25=-m*l*sin(tx)*sin(ty);
m31=m*x*sin(ty);
m32=m*cos(ty)*sin(tx);
m33=m;
m34=0;
m35=0;
m41=-m*l^2*cos(tx)*cos(ty)*sin(ty);
m42=m*l*cos(tx)*cos(ty);
m43=0;
m44=m*l^2*cos(ty)^2;
m45=0;
m51=m*l^2*sin(tx)+m*x*l*cos(ty);
m52=-m*l*sin(tx)*sin(ty);
m53=0;
m54=0;
m55=m*l^2;

c11=bta+m*x*dx+mt*x*dx+m*l*cos(ty)*sin(tx)*dx+m*l*dl-m*l*cos(tx)^2*cos(ty)^2*dl+m*x*cos(ty)*sin(tx)*dl+m*l^2*cos(tx)*cos(ty)^2*sin(tx)*dtx+m*l*x*cos(tx)*cos(ty)*dtx+m*l^2*cos(tx)^2*cos(ty)*sin(ty)*dty-m*x*l*sin(tx)*sin(ty)*dty;
c12=m*x*dta+mt*x*dta+m*l*cos(ty)*sin(tx)*dta;
c13=m*l*dta-m*l*cos(tx)^2*cos(ty)^2*dta+m*x*cos(ty)*sin(ty)*dta-m*l*cos(tx)*cos(ty)*sin(ty)*dtx+m*x*cos(ty)*dty+m*l*sin(tx)*dty;
c14=m*l^2*cos(tx)*cos(ty)^2*sin(ty)*dta+m*x*l*cos(tx)*cos(ty)*dta-m*l*cos(tx)*cos(ty)*sin(ty)*dl+m*l^2*cos(ty)*sin(tx)*sin(ty)*dtx+m*l^2*cos(tx)*dty-m*l^2*cos(tx)*cos(ty)^2*dty;
c15=m*l^2*cos(tx)^2*cos(ty)*sin(ty)*dta-m*x*l*sin(tx)*sin(ty)*dta+m*x*cos(ty)*dl+m*l*sin(tx)*dl+m*l^2*cos(tx)*dtx-m*l^2*cos(tx)*cos(ty)^2*dtx-m*x*l*sin(ty)*dty;
c21=-m*x*dta-mt*x*dta-m*l*cos(ty)*sin(tx)*dta-m*sin(ty)*dl-m*l*cos(ty)*dty;
c22=bx;
c23=-m*sin(ty)*dta+m*cos(tx)*cos(ty)*dtx-m*sin(tx)*sin(ty)*dty;
c24=m*cos(ty)*cos(tx)*dl-m*l*cos(ty)*sin(tx)*dtx-m*l*cos(tx)*sin(ty)*dty;
c25=-m*l*cos(ty)*dta-m*sin(tx)*sin(ty)*dl-m*l*cos(tx)*sin(ty)*dtx-m*l*cos(ty)*sin(tx)*dty;
c31=-m*l*dta+m*l*cos(tx)^2*cos(ty)^2*dta-m*x*cos(ty)*sin(tx)*dta+m*sin(ty)*dx+m*l*cos(tx)*cos(ty)*sin(ty)*dtx-m*l*sin(tx)*dty;
c32=m*sin(ty)*dta;
c33=bl;
c34=m*l*cos(tx)*cos(ty)*sin(ty)*dta-m*l*cos(ty)^2*dtx;
c35=-m*l*sin(tx)*dta-m*l*dty;
c41=-m*l^2*cos(tx)*cos(ty)^2*sin(tx)*dta-m*x*l*cos(tx)*cos(ty)*dta-m*l*cos(tx)*cos(ty)*sin(ty)*dl-m*l^2*cos(tx)*cos(ty)^2*dty;
c42=0;
c43=-m*l*cos(tx)*cos(ty)*sin(ty)*dta+m*l*cos(ty)^2*dtx;
c44=btx+m*l*cos(ty)^2*dl-m*l^2*cos(ty)*sin(ty)*dty;
c45=-m*l^2*cos(tx)*cos(ty)^2*dta-m*l^2*cos(ty)*sin(ty)*dtx;
c51=-m*l^2*cos(tx)^2*cos(ty)*sin(ty)*dta+m*l*x*sin(tx)*sin(ty)*dta+m*l*cos(ty)*dx+m*l*sin(tx)*dl+m*l^2*cos(tx)*cos(ty)^2*dtx;
c52=m*l*cos(ty)*dta;
c53=m*l*dty+m*l*sin(tx)*dta;
c54=m*l^2*cos(tx)*cos(ty)^2*dta+m*l^2*cos(ty)*sin(ty)*dtx;
c55=bty+m*l*dl;

g1=0;
g2=0;
g3=-m*g*cos(tx)*cos(ty);
g4=m*g*l*cos(ty)*sin(tx);
g5=m*g*l*cos(tx)*sin(ty);

M11=[m11 m12 m13;m21 m22 m23;m31 m32 m33];
M12=[m14 m15;m24 m25; m34 m35];
M21=[m41 m42 m43;m51 m52 m53];
M22=[m44 m45;m54 m55];
C11=[c11 c12 c13;c21 c22 c23;c31 c32 c33];
C12=[c14 c15;c24 c25; c34 c35];
C21=[c41 c42 c43;c51 c52 c53];
C22=[c44 c45;c54 c55];

G11=[g1;g2;g3];
G22=[g4;g5];

Mbar = M11 - M12*inv(M22)*M21;
C1bar = C11 - M12*inv(M22)*C21;
C2bar = C12 - M12*inv(M22)*C22;
Gbar = G11 - M12*inv(M22)*G22;

lamda1=0.75;
lamda2=0.5;
lamda3=0.85;
alpha1=0.8;
alpha2=1.8;
lambda = [lamda1 0 0;0 lamda2 0; 0 0 lamda3];
alpha = [alpha1 0;0 alpha2;alpha1/2 alpha2/2];

kappa = 0.2*diag([0.5 0.5 0.5]);

s = e1d + lambda*e1 + alpha*e2;

F = C1bar*dqa + C2bar*dqu + Gbar - kappa*sign(s)- Mbar*(2*lambda*dqa + lambda'*lambda*e1 + alpha*dqu + lambda*alpha*qu);
u=[F(1);F(2);F(3)];
end

== matlab function smceso_simscape/Tower Crane1/MATLAB Function ==
  data: xl2d input; phi output; yl2d input; zl2d input; theta output
function [phi,theta] = calculateangle(xl2d,yl2d,zl2d)
g = 9.81;
phi = atan(-xl2d/(zl2d+g));
mau = sqrt(xl2d^2+(zl2d+g)^2);
theta = atan(yl2d/mau);
end

== matlab function smceso_simscape/MATLAB Function2 ==
  data: xl input; yl input; zl input; ta output; x output; l output; xl2d input; yl2d input; zl2d input
function [ta,x,l] = fcn(xl,yl,zl,xl2d,yl2d,zl2d)
h=45;
g=9.81;
l=(xl2d^2/(g + zl2d)^2 + 1)^(1/2)*(h - zl)*(yl2d^2/((g + zl2d)^2 + xl2d^2) + 1)^(1/2);
x=sqrt(xl^2+yl^2);
ta=-8/300*(l-45);
end
